simulink model "iadc2"  (Simulink 10.0)
settings: Solver=ode45  StartTime=0.0  StopTime=10.0  RelTol=1e-3  EnableMultiTasking=on
values from neighbouring files (symbols this model uses):
  M = OSR    (= 16)    [check_ExCount_dout_9Corner.m]
  OSR = OSR_user    (= 16)    [check_ExCount_dout_9Corner.m]
  tclk = Ts    (= 3.125e-08)    [check_ExCount_dout_9Corner.m]
settings Model: Creator=chench  LastModifiedBy=benve
settings DataIOCC: LimitDataPoints=on  SignalLoggingSaveFormat=ModelDataLogs
settings OptimizationCC: ExpressionDepthLimit=2147483647  InitFltsAndDblsToZero=on
settings DebuggingCC: SaveWithParameterizedLinksMsg=none  SignalResolutionControl=TryResolveAllWithWarning  SolverPrmCheckMsg=warning  MultiTaskDSMMsg=warning  MultiTaskCondExecSysMsg=none  FcnCallInpInsideContextMsg=warning  AllowSymbolicDim=off  StateNameClashWarn=warning
settings GRTTargetCC: TargetFcnLib=ansi_tfl_tmw.mat  GeneratePreprocessorConditionals=Disable all
settings ConfigComp: CovExternalEMLEnable=off

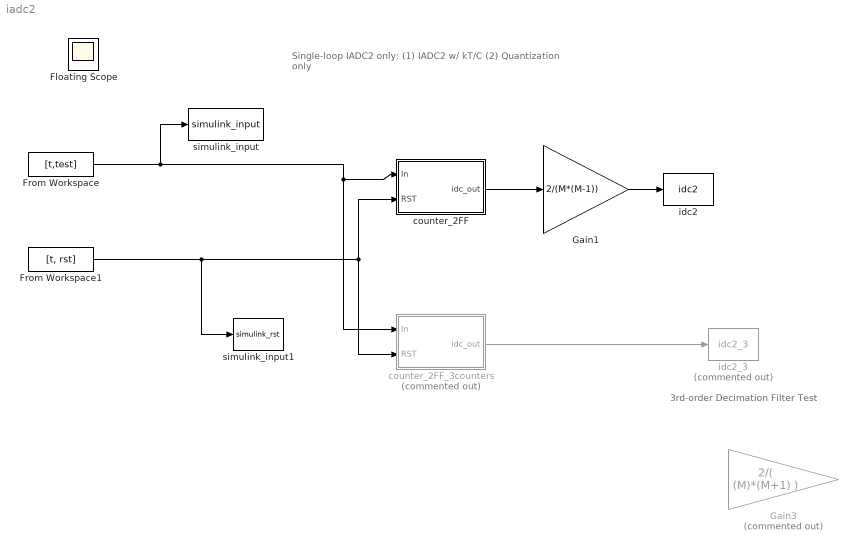
== system iadc2 ==
  note: 3rd-order Decimation Filter Test
  note: Single-loop IADC2 only:
      | (1) IADC2 w/ kT/C (2) Quantization only
  From Workspace : FromWorkspace  VariableName=[t,test]  SampleTime=tclk  Interpolate=off  OutputAfterFinalValue=Holding final value
  From Workspace1 : FromWorkspace  VariableName=[t, rst]  SampleTime=tclk  Interpolate=off  OutputAfterFinalValue=Holding final value
  Gain1 : Gain  Gain=2/(M*(M-1))
  Gain3 : Gain  Commented=on  Gain=2/( (M)*(M+1) )
  counter_2FF : Subsystem
  counter_2FF_3counters : Subsystem  Commented=on
  idc2 : ToWorkspace  VariableName=idc2  SampleTime=-1
  idc2_3 : ToWorkspace  Commented=on  VariableName=idc2_3  SampleTime=-1
  simulink_input : ToWorkspace  VariableName=simulink_input  SampleTime=-1
  simulink_input1 : ToWorkspace  VariableName=simulink_rst  SampleTime=-1
  Floating Scope : Scope
  wires:
  From Workspace1/1 -> simulink_input1/1, counter_2FF_3counters/2(RST), counter_2FF/2(RST)
  From Workspace/1 -> counter_2FF/1(In), counter_2FF_3counters/1(In), simulink_input/1
  counter_2FF_3counters/1(idc_out) -> idc2_3/1
  counter_2FF/1(idc_out) -> Gain1/1
  Gain1/1 -> idc2/1

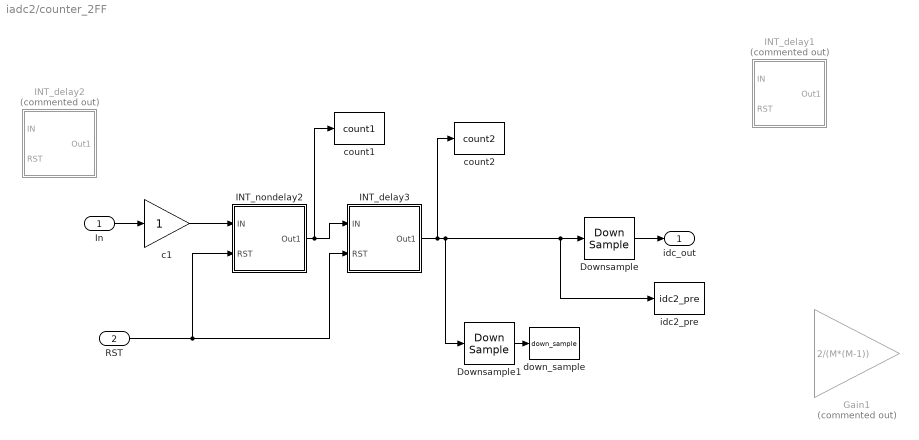
== system iadc2/counter_2FF ==
  In : Inport
  RST : Inport  Port=2
  Downsample : DownSample  N=OSR  phase=OSR-1  RateOptions=Allow multirate processing
  Downsample1 : DownSample  N=OSR  phase=OSR-1  RateOptions=Allow multirate processing
  Gain1 : Gain  Commented=on  Gain=2/(M*(M-1))
  INT_delay1 : Subsystem  Commented=on
  INT_delay2 : Subsystem  Commented=on
  INT_delay3 : Subsystem
  INT_nondelay2 : Subsystem
  c1 : Gain  SaturateOnIntegerOverflow=on  OutDataTypeStr=Inherit: Same as input  ParamDataTypeStr=Inherit: Same as input
  count1 : ToWorkspace  VariableName=count1  SampleTime=-1
  count2 : ToWorkspace  VariableName=count2  SampleTime=-1
  down_sample : ToWorkspace  VariableName=down_sample  SampleTime=-1
  "idc2_pre " : ToWorkspace  VariableName=idc2_pre  SampleTime=-1
  idc_out : Outport  VectorParamsAs1DForOutWhenUnconnected=off
  wires:
  RST/1 -> INT_nondelay2/2(RST), INT_delay3/2(RST)
  Downsample/1 -> idc_out/1
  In/1 -> c1/1
  INT_delay3/1(Out1) -> count2/1, "idc2_pre "/1, Downsample/1, Downsample1/1
  INT_nondelay2/1(Out1) -> count1/1, INT_delay3/1(IN)
  c1/1 -> INT_nondelay2/1(IN)
  Downsample1/1 -> down_sample/1

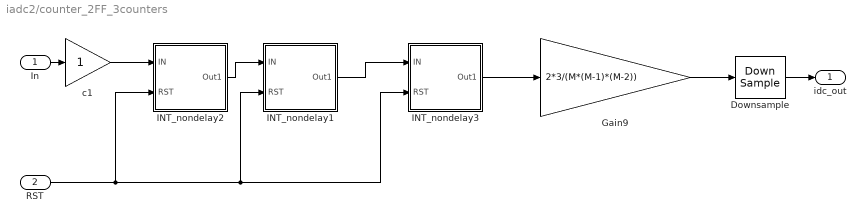
== system iadc2/counter_2FF_3counters ==
  In : Inport
  RST : Inport  Port=2
  Downsample : DownSample  N=OSR  phase=OSR-1  RateOptions=Allow multirate processing
  Gain9 : Gain  Gain=2*3/(M*(M-1)*(M-2))
  INT_nondelay1 : Subsystem
  INT_nondelay2 : Subsystem
  INT_nondelay3 : Subsystem
  c1 : Gain  SaturateOnIntegerOverflow=on  OutDataTypeStr=Inherit: Same as input  ParamDataTypeStr=Inherit: Same as input
  idc_out : Outport  VectorParamsAs1DForOutWhenUnconnected=off
  wires:
  RST/1 -> INT_nondelay3/2(RST), INT_nondelay1/2(RST), INT_nondelay2/2(RST)
  Downsample/1 -> idc_out/1
  c1/1 -> INT_nondelay2/1(IN)
  In/1 -> c1/1
  INT_nondelay2/1(Out1) -> INT_nondelay1/1(IN)
  INT_nondelay1/1(Out1) -> INT_nondelay3/1(IN)
  INT_nondelay3/1(Out1) -> Gain9/1
  Gain9/1 -> Downsample/1

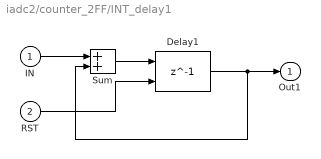
== system iadc2/counter_2FF/INT_delay1 ==
  IN : Inport
  RST : Inport  Port=2
  Delay1 : Delay  DelayLength=1  InitialCondition=0  ExternalReset=Rising
      settings: InputPortMap=u0,r5
  Sum : Sum  SaturateOnIntegerOverflow=on  InputSameDT=on  OutDataTypeStr=Inherit: Same as first input
  Out1 : Outport  VectorParamsAs1DForOutWhenUnconnected=off
  wires:
  IN/1 -> Sum/1
  Sum/1 -> Delay1/1
  Delay1/1 -> Sum/2, Out1/1
  RST/1 -> Delay1/2

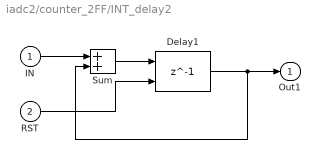
== system iadc2/counter_2FF/INT_delay2 ==
  IN : Inport
  RST : Inport  Port=2
  Delay1 : Delay  DelayLength=1  InitialCondition=0  ExternalReset=Rising
      settings: InputPortMap=u0,r5
  Sum : Sum  SaturateOnIntegerOverflow=on  InputSameDT=on  OutDataTypeStr=Inherit: Same as first input
  Out1 : Outport  VectorParamsAs1DForOutWhenUnconnected=off
  wires:
  IN/1 -> Sum/1
  Sum/1 -> Delay1/1
  Delay1/1 -> Sum/2, Out1/1
  RST/1 -> Delay1/2

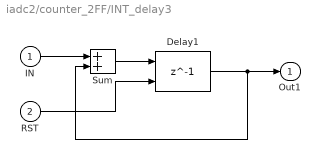
== system iadc2/counter_2FF/INT_delay3 ==
  IN : Inport
  RST : Inport  Port=2
  Delay1 : Delay  DelayLength=1  InitialCondition=0  ExternalReset=Rising
      settings: InputPortMap=u0,r5
  Sum : Sum  SaturateOnIntegerOverflow=on  InputSameDT=on  OutDataTypeStr=Inherit: Same as first input
  Out1 : Outport  VectorParamsAs1DForOutWhenUnconnected=off
  wires:
  IN/1 -> Sum/1
  Sum/1 -> Delay1/1
  Delay1/1 -> Sum/2, Out1/1
  RST/1 -> Delay1/2

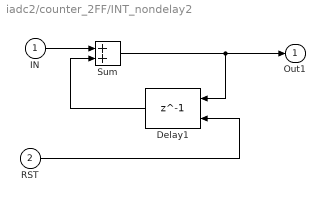
== system iadc2/counter_2FF/INT_nondelay2 ==
  IN : Inport
  RST : Inport  Port=2
  Delay1 : Delay  DelayLength=1  InitialCondition=0  ExternalReset=Rising
      settings: InputPortMap=u0,r5
  Sum : Sum  SaturateOnIntegerOverflow=on  InputSameDT=on  OutDataTypeStr=Inherit: Same as first input
  Out1 : Outport  VectorParamsAs1DForOutWhenUnconnected=off
  wires:
  IN/1 -> Sum/1
  Sum/1 -> Delay1/1, Out1/1
  RST/1 -> Delay1/2
  Delay1/1 -> Sum/2

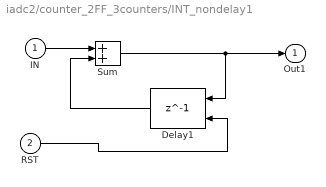
== system iadc2/counter_2FF_3counters/INT_nondelay1 ==
  IN : Inport
  RST : Inport  Port=2
  Delay1 : Delay  DelayLength=1  InitialCondition=0  ExternalReset=Rising
      settings: InputPortMap=u0,r5
  Sum : Sum  SaturateOnIntegerOverflow=on  InputSameDT=on  OutDataTypeStr=Inherit: Same as first input
  Out1 : Outport  VectorParamsAs1DForOutWhenUnconnected=off
  wires:
  IN/1 -> Sum/1
  Sum/1 -> Delay1/1, Out1/1
  RST/1 -> Delay1/2
  Delay1/1 -> Sum/2

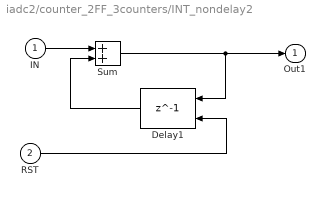
== system iadc2/counter_2FF_3counters/INT_nondelay2 ==
  IN : Inport
  RST : Inport  Port=2
  Delay1 : Delay  DelayLength=1  InitialCondition=0  ExternalReset=Rising
      settings: InputPortMap=u0,r5
  Sum : Sum  SaturateOnIntegerOverflow=on  InputSameDT=on  OutDataTypeStr=Inherit: Same as first input
  Out1 : Outport  VectorParamsAs1DForOutWhenUnconnected=off
  wires:
  IN/1 -> Sum/1
  Sum/1 -> Delay1/1, Out1/1
  RST/1 -> Delay1/2
  Delay1/1 -> Sum/2

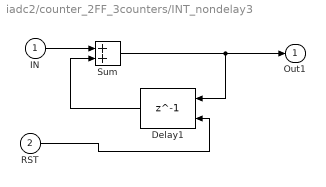
== system iadc2/counter_2FF_3counters/INT_nondelay3 ==
  IN : Inport
  RST : Inport  Port=2
  Delay1 : Delay  DelayLength=1  InitialCondition=0  ExternalReset=Rising
      settings: InputPortMap=u0,r5
  Sum : Sum  SaturateOnIntegerOverflow=on  InputSameDT=on  OutDataTypeStr=Inherit: Same as first input
  Out1 : Outport  VectorParamsAs1DForOutWhenUnconnected=off
  wires:
  IN/1 -> Sum/1
  Sum/1 -> Delay1/1, Out1/1
  RST/1 -> Delay1/2
  Delay1/1 -> Sum/2
